simulink model "AtomsModel"  (R2024a)
settings: Solver=FixedStepDiscrete  StartTime=0.0  StopTime=10.0  RelTol=1e-3
settings Model: Creator=BIDO  LastModifiedBy=BIDO
settings OptimizationCC: DefaultParameterBehavior=Inlined  UseDivisionForNetSlopeComputation=on  GainParamInheritBuiltInType=on  UseFloatMulNetSlope=on  InlineInvariantSignals=on  EnhancedBackFolding=on  PassReuseOutputArgsAs=Individual arguments  ZeroExternalMemoryAtStartup=off  ZeroInternalMemoryAtStartup=off  NoFixptDivByZeroProtection=on  EfficientFloat2IntCast=on  LifeSpan=1  OptimizeBlockOrder=speed  DifferentSizesBufferReuse=on  OptimizationCustomize=off  EfficientTunableParamExpr=on
settings DebuggingCC: ParameterTunabilityLossMsg=error
settings HardwareCC: ProdLongLongMode=on
settings SFSimCC: MATLABDynamicMemAlloc=off
settings RTWCC: Description=Embedded Coder  SystemTargetFile=ert.tlc  TemplateMakefile=ert_default_tmf
settings CodeAppCC: ForceParamTrailComments=on  IgnoreCustomStorageClasses=off  MaxIdLength=50  OperatorAnnotations=on  SimulinkDataObjDesc=on  SFDataObjDesc=on  MangleLength=2  CustomSymbolStrGlobalVar=$R$N$M_Global_var  CustomSymbolStrType=$N$R$M__Global_struct  CustomSymbolStrFcn=GAZA_$N$M$F  CustomSymbolStrFcnArg=FreePalestine_$I$N$M  InsertBlockDesc=on  InternalIdentifier=Classic
settings ERTTargetCC: TargetLangStandard=C99 (ISO)  GenerateSampleERTMain=on  IncludeMdlTerminateFcn=off  CombineSignalStateStructs=on  SuppressErrorStatus=on  SupportAbsoluteTime=off  SupportComplex=off  InlinedParameterPlacement=NonHierarchical  ERTCustomFileTemplate=example_file_process.tlc

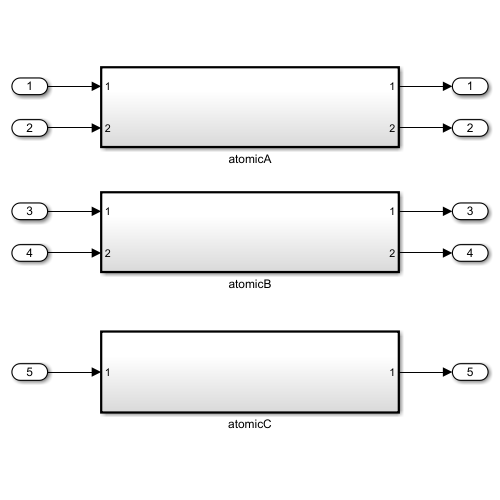
[thumbnail: Simulink's stored preview of the top-level diagram]
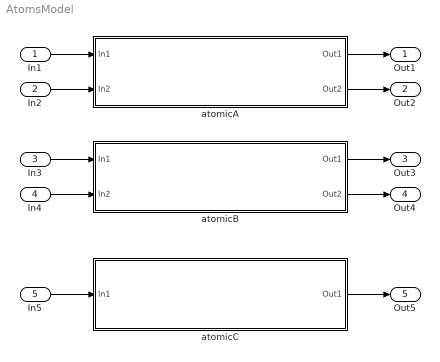
== system AtomsModel ==
  In1 : Inport
  In2 : Inport  Port=2
  In3 : Inport  Port=3
  In4 : Inport  Port=4
  In5 : Inport  Port=5
  atomicA : Subsystem  TreatAsAtomicUnit=on  RTWFcnName=myAtomicFuncA
      settings: RTWSystemCode=Nonreusable function  RTWFcnNameOpts=User specified
  atomicB : Subsystem  TreatAsAtomicUnit=on
      settings: RTWSystemCode=Nonreusable function  FunctionInterfaceSpec=Allow arguments (Optimized)
  atomicC : Subsystem  TreatAsAtomicUnit=on
      settings: RTWSystemCode=Nonreusable function  FunctionInterfaceSpec=Allow arguments (Match graphical interface)
  Out1 : Outport
  Out2 : Outport  Port=2
  Out3 : Outport  Port=3
  Out4 : Outport  Port=4
  Out5 : Outport  Port=5
  wires:
  atomicA/1(Out1) -> Out1/1
  atomicA/2(Out2) -> Out2/1
  In2/1 -> atomicA/2(In2)
  In1/1 -> atomicA/1(In1)
  In3/1 -> atomicB/1(In1)
  In4/1 -> atomicB/2(In2)
  atomicB/2(Out2) -> Out4/1
  atomicB/1(Out1) -> Out3/1
  atomicC/1(Out1) -> Out5/1
  In5/1 -> atomicC/1(In1)

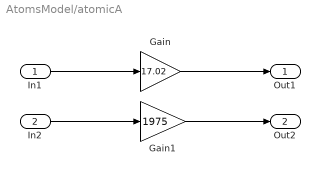
== system AtomsModel/atomicA ==
  In1 : Inport
  In2 : Inport  Port=2
  Gain : Gain  Gain=17.02
  Gain1 : Gain  Gain=1975
  Out1 : Outport
  Out2 : Outport  Port=2
  wires:
  Gain/1 -> Out1/1
  In1/1 -> Gain/1
  In2/1 -> Gain1/1
  Gain1/1 -> Out2/1

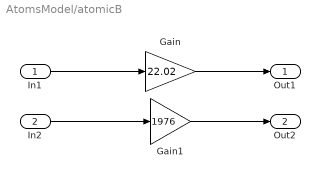
== system AtomsModel/atomicB ==
  In1 : Inport
  In2 : Inport  Port=2
  Gain : Gain  Gain=22.02
  Gain1 : Gain  Gain=1976
  Out1 : Outport
  Out2 : Outport  Port=2
  wires:
  Gain1/1 -> Out2/1
  In2/1 -> Gain1/1
  In1/1 -> Gain/1
  Gain/1 -> Out1/1

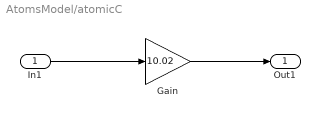
== system AtomsModel/atomicC ==
  In1 : Inport
  Gain : Gain  Gain=10.02
  Out1 : Outport
  wires:
  Gain/1 -> Out1/1
  In1/1 -> Gain/1
